simulink library "libc_parts_valves"  (R2015b)
settings: Solver=FixedStepDiscrete  StartTime=0.0  StopTime=Inf  FixedStep=0.004  RelTol=1e-3
PostLoadFcn:
  | , if any(exist('dsrtsu_mdlpostloadfcn', 'file') == [2, 3, 6]), try dsrtsu_mdlpostloadfcn('Execute', bdroot); catch fprintf('Error in PostLoadFcn (dsrtsu_mdlpostloadfcn) for model "%s":\n %s\n', bdroot, lasterr); end, end,
undefined symbols (not defined in the file or in its folder): den, num
undefined symbols (not defined in the file): tA
libraries: libc_parts_valves x9, simulink x6, libc_extended_basics x2, PMC_lib x1
settings Model: DSRTSU_INTERNAL_RTI_VER=470  DSRTSU_INTERNAL_RTI_TYPE=rti1007  DSRTSU_INTERNAL_RTIFPGA=60  Creator=Falkenhahn  LastModifiedBy=Falkenhahn
settings DataIOCC: SaveFormat=Array
settings OptimizationCC: BlockReduction=off  OptimizeBlockIOStorage=off  BufferReuse=off  GlobalBufferReuse=off  ExpressionFolding=off  LocalBlockOutputs=off
settings DebuggingCC: UnderspecifiedInitializationDetection=Classic  MergeDetectMultiDrivingBlocksExec=none  SolverPrmCheckMsg=warning
settings HardwareCC: ProdBitPerPointer=32  ProdLargestAtomicFloat=None  ProdEndianess=BigEndian  ProdWordSize=32  ProdHWDeviceType=Generic->Custom  TargetIntDivRoundTo=Zero  TargetEndianess=BigEndian  TargetHWDeviceType=Generic->Custom
settings RTWCC: SystemTargetFile=rti1007.tlc  MakeCommand=make_rti  TemplateMakefile=rti1007.tmf  Description=dSPACE DS1007 Hardware Platform
settings STFCustomTargetCC: ParMdlRefBuildCompliant=on  ConcurrentExecutionCompliant=off  MatFileLogging=on  SystemTargetFile=rti1007.tlc
settings GRTTargetCC: CompOptLevelCompliant=off  ConcurrentExecutionCompliant=off  GeneratePreprocessorConditionals=Disable all  CombineOutputUpdateFcns=off  GRTInterface=on  UseToolchainInfoCompliant=off  ExtModeMexFile=noextcomm
settings ConfigComp: CovModelRefEnable=Off

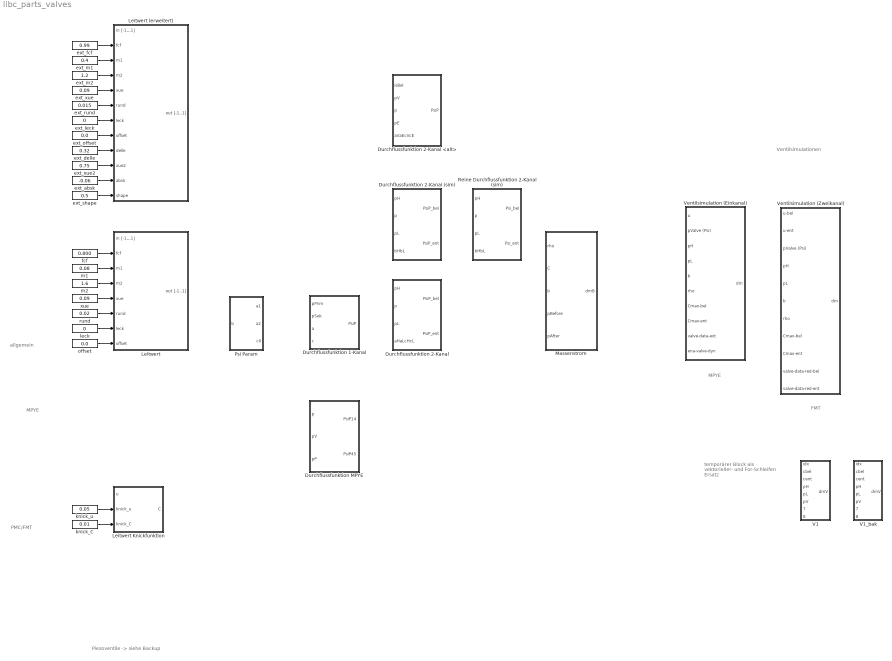
== system libc_parts_valves ==
  note: temporärer Block als
      | vektorieller- und For-Schleifen
      | Ersatz
  note: MPYE
  note: allgemein
  note: MPYE
  note: Piezoventile -> siehe Backup
  note: PMC/FMT
  note: Ventilsimulationen
  note: FMT
  Durchflussfunktion 1-Kanal : Subsystem
      settings: AttributesFormatString=gebrochenrational
  Durchflussfunktion 2-Kanal : Subsystem
      settings: AttributesFormatString=gebrochenrational
  Durchflussfunktion 2-Kanal (sim) : Subsystem
      settings: AttributesFormatString=|
      | Wurzelfunktion
      | (nicht geeignet für Ventilinvertierung)
  Durchflussfunktion 2-Kanal <alt> : Subsystem
      settings: AttributesFormatString=gebrochenrational
  Durchflussfunktion MPYE : Subsystem
      settings: AttributesFormatString=|
      | gebrochenrational
      | kanalweise mit b=0.3
  Leitwert : Subsystem  mask{invertcomp=on}
      mask prompts: invertcomp "Invertierter Leitwert"
      mask help: Leitwertberechnung
      settings: AttributesFormatString=|
      | inv: Cn --> u (on)
      | hin: u --> Cn (off)
      | Invertiert: %<invertcomp>
  Leitwert (erweitert) : Subsystem  mask{invertcomp=on}
      mask prompts: invertcomp "Invertierter Leitwert"
      mask help: Leitwertberechnung
      settings: AttributesFormatString=|
      | inv: Cn --> u (on)
      | hin: u --> Cn (off)
      | Invertiert: %<invertcomp>
  Leitwert Knickfunktion : MATLAB Function  TreatAsAtomicUnit=on
      settings: AttributesFormatString=|
      | u (0..1) -> C (0..1)
      | vertausche knick_u
      | und knick_C-Parameter
      | zur Berechnung der
      | Invertierung
  Massenstrom : Subsystem
  Psi Param : Subsystem
      settings: AttributesFormatString=sqrt -> geb-rat
  Reine Durchflussfunktion 2-Kanal (sim) : Subsystem
      settings: AttributesFormatString=Wurzelfunktion
  V1 : Subsystem
  V1_bak : Subsystem
  Ventilsimulation (Einkanal) : Subsystem
      settings: AttributesFormatString=|
      | mit Wurzelfunktion
      | nicht für Invertierung geeignet
  Ventilsimulation (Zweikanal) : Subsystem
      settings: AttributesFormatString=|
      | mit Wurzelfunktion
      | nicht für Invertierung geeignet
      | 2-Kanal (reduzierte valve-data, ohne valve_dyn)
  ext_absk : Constant  Value=-0.06
  ext_delle : Constant  Value=0.32
  ext_fcf : Constant  Value=0.99
  ext_leck : Constant  Value=0
  ext_m1 : Constant  Value=0.4
  ext_m2 : Constant  Value=1.2
  ext_offset : Constant  Value=0.0
  ext_rund : Constant  Value=0.015
  ext_shape : Constant  Value=0.5
  ext_xue : Constant  Value=0.09
  ext_xue2 : Constant  Value=0.75
  fcf : Constant  Value=0.800
  knick_C : Constant  Value=0.01
  knick_u : Constant  Value=0.05
  leck : Constant  Value=0
  m1 : Constant  Value=0.08
  m2 : Constant  Value=1.6
  offset : Constant  Value=0.0
  rund : Constant  Value=0.02
  xue : Constant  Value=0.09
  wires:
  m1/1 -> Leitwert/3(m1)
  fcf/1 -> Leitwert/2(fcf)
  offset/1 -> Leitwert/8(offset)
  rund/1 -> Leitwert/6(rund)
  m2/1 -> Leitwert/4(m2)
  xue/1 -> Leitwert/5(xue)
  leck/1 -> Leitwert/7(leck)
  ext_m1/1 -> Leitwert (erweitert)/3(m1)
  ext_fcf/1 -> Leitwert (erweitert)/2(fcf)
  ext_offset/1 -> Leitwert (erweitert)/8(offset)
  ext_rund/1 -> Leitwert (erweitert)/6(rund)
  ext_m2/1 -> Leitwert (erweitert)/4(m2)
  ext_xue/1 -> Leitwert (erweitert)/5(xue)
  ext_leck/1 -> Leitwert (erweitert)/7(leck)
  ext_delle/1 -> Leitwert (erweitert)/9(delle)
  ext_xue2/1 -> Leitwert (erweitert)/10(xue2)
  ext_absk/1 -> Leitwert (erweitert)/11(absk)
  ext_shape/1 -> Leitwert (erweitert)/12(shape)
  knick_u/1 -> Leitwert Knickfunktion/2(knick_u)
  knick_C/1 -> Leitwert Knickfunktion/3(knick_C)

== system libc_parts_valves/Durchflussfunktion 1-Kanal ==
  pPrim : Inport
  pSek : Inport  Port=2
  a : Inport  Port=3
  c : Inport  Port=4
  Durchflussfunktion 1 : MATLAB Function  TreatAsAtomicUnit=on
      settings: AttributesFormatString=gebrochenrational
  PsiP : Outport
  wires:
  pSek/1 -> Durchflussfunktion 1/2(pSek)
  a/1 -> Durchflussfunktion 1/3(a)
  pPrim/1 -> Durchflussfunktion 1/1(pPrim)
  Durchflussfunktion 1/1(PsiP) -> PsiP/1
  c/1 -> Durchflussfunktion 1/4(c)

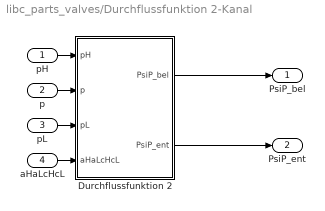
== system libc_parts_valves/Durchflussfunktion 2-Kanal ==
  pH : Inport
  p : Inport  Port=2
  pL : Inport  Port=3
  aHaLcHcL : Inport  Port=4
  Durchflussfunktion 2 : MATLAB Function  TreatAsAtomicUnit=on
      settings: AttributesFormatString=gebrochenrational
  PsiP_bel : Outport
  PsiP_ent : Outport  Port=2
  wires:
  pH/1 -> Durchflussfunktion 2/1(pH)
  pL/1 -> Durchflussfunktion 2/3(pL)
  p/1 -> Durchflussfunktion 2/2(p)
  aHaLcHcL/1 -> Durchflussfunktion 2/4(aHaLcHcL)
  Durchflussfunktion 2/1(PsiP_bel) -> PsiP_bel/1
  Durchflussfunktion 2/2(PsiP_ent) -> PsiP_ent/1

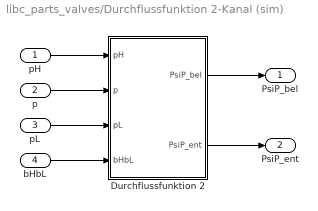
== system libc_parts_valves/Durchflussfunktion 2-Kanal (sim) ==
  pH : Inport
  p : Inport  Port=2
  pL : Inport  Port=3
  bHbL : Inport  Port=4
  Durchflussfunktion 2 : MATLAB Function  TreatAsAtomicUnit=on
      settings: AttributesFormatString=Wurzelfunktion
  PsiP_bel : Outport
  PsiP_ent : Outport  Port=2
  wires:
  Durchflussfunktion 2/2(PsiP_ent) -> PsiP_ent/1
  Durchflussfunktion 2/1(PsiP_bel) -> PsiP_bel/1
  bHbL/1 -> Durchflussfunktion 2/4(bHbL)
  p/1 -> Durchflussfunktion 2/2(p)
  pL/1 -> Durchflussfunktion 2/3(pL)
  pH/1 -> Durchflussfunktion 2/1(pH)

== system libc_parts_valves/Durchflussfunktion 2-Kanal <alt> ==
  isBel : Inport
  pV : Inport  Port=2
  p : Inport  Port=3
  pE : Inport  Port=4
  aVaEcVcE : Inport  Port=5
  Durchflussfunktion 2 : MATLAB Function  TreatAsAtomicUnit=on
      settings: AttributesFormatString=gebrochenrational
  PsiP : Outport
  wires:
  isBel/1 -> Durchflussfunktion 2/1(isBel)
  pV/1 -> Durchflussfunktion 2/2(pV)
  pE/1 -> Durchflussfunktion 2/4(pE)
  p/1 -> Durchflussfunktion 2/3(p)
  aVaEcVcE/1 -> Durchflussfunktion 2/5(aVaEcVcE)
  Durchflussfunktion 2/1(PsiP) -> PsiP/1

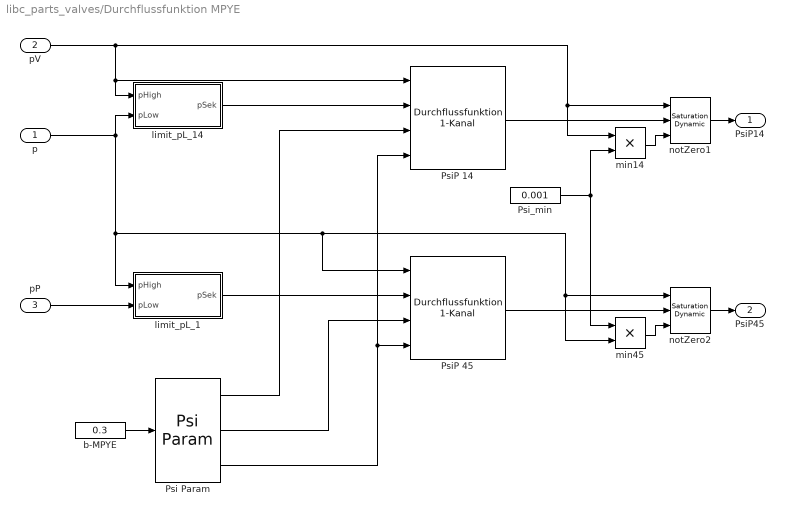
== system libc_parts_valves/Durchflussfunktion MPYE ==
  p : Inport
  pV : Inport  Port=2
  pP : Inport  Port=3
  Psi Param : libc_parts_valves/Psi Param
      settings: AttributesFormatString=sqrt -> geb-rat
  PsiP 14 : libc_parts_valves/Durchflussfunktion 1-Kanal
      settings: AttributesFormatString=gebrochenrational
  PsiP 45 : libc_parts_valves/Durchflussfunktion 1-Kanal
      settings: AttributesFormatString=gebrochenrational
  Psi_min : Constant  Value=0.001
  b-MPYE : Constant  Value=0.3
  limit_pL_1 : MATLAB Function  TreatAsAtomicUnit=on
  limit_pL_14 : MATLAB Function  TreatAsAtomicUnit=on
  min14 : Product  RndMeth=Zero
  min45 : Product  RndMeth=Zero
  notZero1 : simulink/Discontinuities/Saturation Dynamic  OutMin=[]  OutMax=[]  OutDataTypeStr=Inherit: Same as second input  OutDataType=fixdt(1, 16)  OutScaling=2^-10  DoSatur=off
  notZero2 : simulink/Discontinuities/Saturation Dynamic  OutMin=[]  OutMax=[]  OutDataTypeStr=Inherit: Same as second input  OutDataType=fixdt(1, 16)  OutScaling=2^-10  DoSatur=off
  PsiP14 : Outport
  PsiP45 : Outport  Port=2
  wires:
  Psi_min/1 -> min45/1, min14/2
  min45/1 -> notZero2/3
  min14/1 -> notZero1/3
  notZero2/1 -> PsiP45/1
  PsiP 45/1 -> notZero2/2
  notZero1/1 -> PsiP14/1
  PsiP 14/1 -> notZero1/2
  limit_pL_1/1(pSek) -> PsiP 45/2
  limit_pL_14/1(pSek) -> PsiP 14/2
  p/1 -> limit_pL_1/1(pHigh), PsiP 45/1, notZero2/1, min45/2, limit_pL_14/2(pLow)
  pP/1 -> limit_pL_1/2(pLow)
  pV/1 -> notZero1/1, min14/1, PsiP 14/1, limit_pL_14/1(pHigh)
  Psi Param/1 -> PsiP 14/3
  Psi Param/2 -> PsiP 45/3
  Psi Param/3 -> PsiP 14/4, PsiP 45/4
  b-MPYE/1 -> Psi Param/1

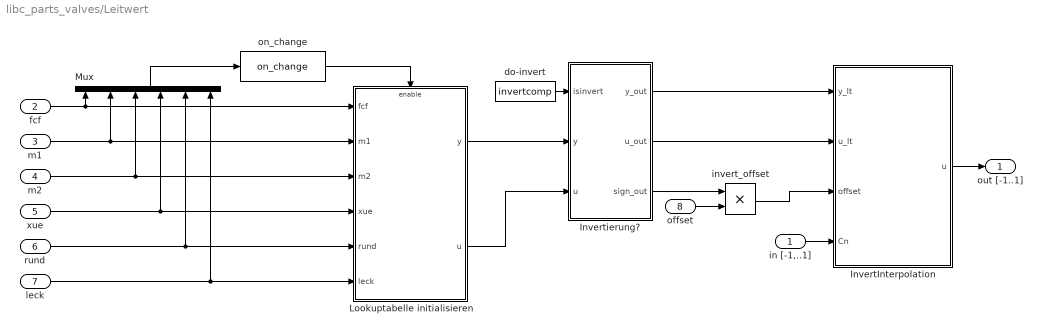
== system libc_parts_valves/Leitwert ==
  in [-1,..1] : Inport
  fcf : Inport  Port=2
  m1 : Inport  Port=3
  m2 : Inport  Port=4
  xue : Inport  Port=5
  rund : Inport  Port=6
  leck : Inport  Port=7
  offset : Inport  Port=8
  InvertInterpolation : MATLAB Function  TreatAsAtomicUnit=on
      settings: AttributesFormatString=|
      | 2 Versionen:
      | alt (PLC-kompatibel)
      | neu (interp1)
  Invertierung? : MATLAB Function  TreatAsAtomicUnit=on
  Lookuptabelle initialisieren : Subsystem  TreatAsAtomicUnit=on
      settings: AttributesFormatString=|
      | 2 Versionen:
      | alt (PLC-kompatibel, mit/ohne Fehler)
      | neu (schnell)
  Mux : Mux  Inputs=6
  do-invert : Constant  Value=invertcomp
  invert_offset : Product
  on_change : libc_extended_basics/on_change  IC=-1
  out [-1..1] : Outport
  wires:
  leck/1 -> Mux/6, Lookuptabelle initialisieren/6(leck)
  Lookuptabelle initialisieren/2(u) -> Invertierung?/3(u)
  offset/1 -> invert_offset/2
  m1/1 -> Mux/2, Lookuptabelle initialisieren/2(m1)
  m2/1 -> Mux/3, Lookuptabelle initialisieren/3(m2)
  rund/1 -> Mux/5, Lookuptabelle initialisieren/5(rund)
  xue/1 -> Mux/4, Lookuptabelle initialisieren/4(xue)
  Lookuptabelle initialisieren/1(y) -> Invertierung?/2(y)
  fcf/1 -> Mux/1, Lookuptabelle initialisieren/1(fcf)
  InvertInterpolation/1(u) -> out [-1..1]/1
  in [-1,..1]/1 -> InvertInterpolation/4(Cn)
  on_change/1 -> Lookuptabelle initialisieren/Enable
  Mux/1 -> on_change/1
  Invertierung?/2(u_out) -> InvertInterpolation/2(u_lt)
  Invertierung?/1(y_out) -> InvertInterpolation/1(y_lt)
  invert_offset/1 -> InvertInterpolation/3(offset)
  Invertierung?/3(sign_out) -> invert_offset/1
  do-invert/1 -> Invertierung?/1(isinvert)

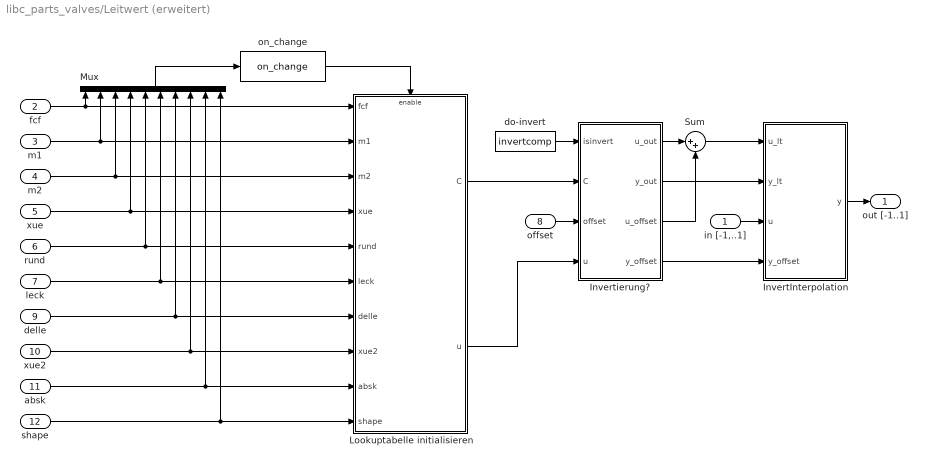
== system libc_parts_valves/Leitwert (erweitert) ==
  in [-1,..1] : Inport
  fcf : Inport  Port=2
  m1 : Inport  Port=3
  m2 : Inport  Port=4
  xue : Inport  Port=5
  rund : Inport  Port=6
  leck : Inport  Port=7
  offset : Inport  Port=8
  delle : Inport  Port=9
  xue2 : Inport  Port=10
  absk : Inport  Port=11
  shape : Inport  Port=12
  InvertInterpolation : MATLAB Function  TreatAsAtomicUnit=on
      settings: AttributesFormatString=|
      | 2 Versionen:
      | alt (PLC-kompatibel)
      | neu (interp1)
  Invertierung? : MATLAB Function  TreatAsAtomicUnit=on
  Lookuptabelle initialisieren : Subsystem  TreatAsAtomicUnit=on
      settings: AttributesFormatString=|
      | 2 Versionen:
      | alt (PLC-kompatibel, mit/ohne Fehler)
      | neu (schnell)
  Mux : Mux  Inputs=10
  Sum : Sum  Inputs=|++
  do-invert : Constant  Value=invertcomp
  on_change : libc_extended_basics/on_change  IC=-1
  out [-1..1] : Outport
  wires:
  Invertierung?/4(y_offset) -> InvertInterpolation/4(y_offset)
  Lookuptabelle initialisieren/2(u) -> Invertierung?/4(u)
  Lookuptabelle initialisieren/1(C) -> Invertierung?/2(C)
  shape/1 -> Lookuptabelle initialisieren/10(shape), Mux/10
  absk/1 -> Lookuptabelle initialisieren/9(absk), Mux/9
  xue2/1 -> Lookuptabelle initialisieren/8(xue2), Mux/8
  delle/1 -> Lookuptabelle initialisieren/7(delle), Mux/7
  leck/1 -> Lookuptabelle initialisieren/6(leck), Mux/6
  offset/1 -> Invertierung?/3(offset)
  m1/1 -> Lookuptabelle initialisieren/2(m1), Mux/2
  m2/1 -> Lookuptabelle initialisieren/3(m2), Mux/3
  rund/1 -> Lookuptabelle initialisieren/5(rund), Mux/5
  xue/1 -> Lookuptabelle initialisieren/4(xue), Mux/4
  fcf/1 -> Mux/1, Lookuptabelle initialisieren/1(fcf)
  in [-1,..1]/1 -> InvertInterpolation/3(u)
  on_change/1 -> Lookuptabelle initialisieren/Enable
  Mux/1 -> on_change/1
  do-invert/1 -> Invertierung?/1(isinvert)
  Invertierung?/1(u_out) -> Sum/1
  Sum/1 -> InvertInterpolation/1(u_lt)
  Invertierung?/2(y_out) -> InvertInterpolation/2(y_lt)
  Invertierung?/3(u_offset) -> Sum/2
  InvertInterpolation/1(y) -> out [-1..1]/1

== system libc_parts_valves/Massenstrom ==
  rho : Inport
  C : Inport  Port=2
  b : Inport  Port=3
  pBefore : Inport  Port=4
  pAfter : Inport  Port=5
  Massenstrom : MATLAB Function  TreatAsAtomicUnit=on
  dmB : Outport
  wires:
  pBefore/1 -> Massenstrom/4(pBefore)
  pAfter/1 -> Massenstrom/5(pAfter)
  C/1 -> Massenstrom/2(parC)
  b/1 -> Massenstrom/3(parb)
  Massenstrom/1(mBdot) -> dmB/1
  rho/1 -> Massenstrom/1(parrho)

== system libc_parts_valves/Psi Param ==
  b : Inport
  b-auto : MATLAB Function  TreatAsAtomicUnit=on
  a1 : Outport
  a2 : Outport  Port=2
  c0 : Outport  Port=3
  wires:
  b/1 -> b-auto/1(b)
  b-auto/1(a1) -> a1/1
  b-auto/3(c0) -> c0/1
  b-auto/2(a2) -> a2/1

== system libc_parts_valves/Reine Durchflussfunktion 2-Kanal (sim) ==
  pH : Inport
  p : Inport  Port=2
  pL : Inport  Port=3
  bHbL : Inport  Port=4
  Durchflussfunktion 2 : MATLAB Function  TreatAsAtomicUnit=on
      settings: AttributesFormatString=Wurzelfunktion
  Psi_bel : Outport
  Psi_ent : Outport  Port=2
  wires:
  pH/1 -> Durchflussfunktion 2/1(pH)
  pL/1 -> Durchflussfunktion 2/3(pL)
  p/1 -> Durchflussfunktion 2/2(p)
  bHbL/1 -> Durchflussfunktion 2/4(bHbL)
  Durchflussfunktion 2/1(Psi_bel) -> Psi_bel/1
  Durchflussfunktion 2/2(Psi_ent) -> Psi_ent/1

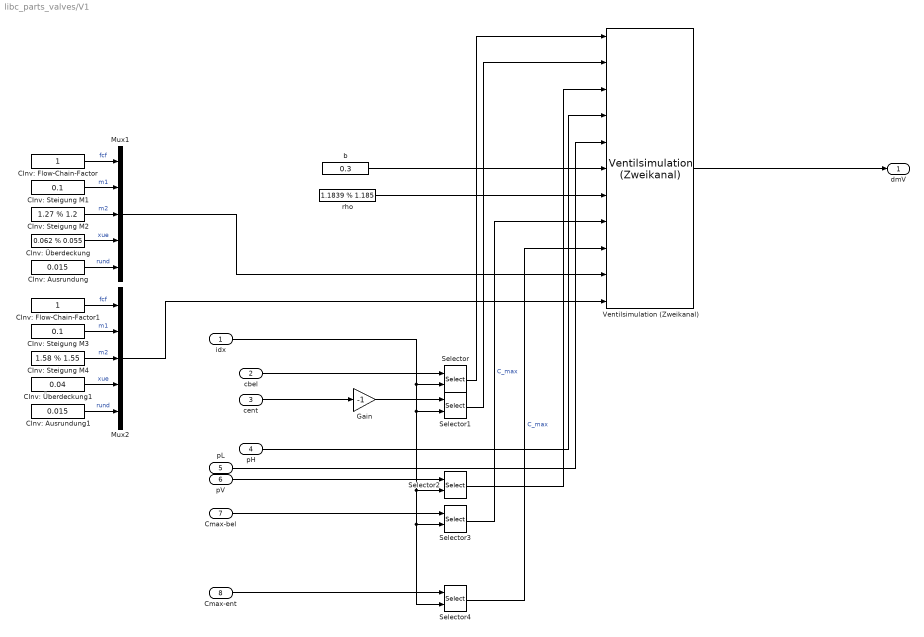
== system libc_parts_valves/V1 ==
  idx : Inport
  cbel : Inport  Port=2
  cent : Inport  Port=3
  pH : Inport  Port=4
  pL : Inport  Port=5
  pV : Inport  Port=6
  Cmax-bel : Inport  Port=7
  Cmax-ent : Inport  Port=8
  CInv: Ausrundung : Constant  Value=0.015
  CInv: Ausrundung1 : Constant  Value=0.015
  CInv: Flow-Chain-Factor : Constant
  CInv: Flow-Chain-Factor1 : Constant
  CInv: Steigung M1 : Constant  Value=0.1
  CInv: Steigung M2 : Constant  Value=1.27 % 1.2
  CInv: Steigung M3 : Constant  Value=0.1
  CInv: Steigung M4 : Constant  Value=1.58 % 1.55
  CInv: Überdeckung : Constant  Value=0.062 % 0.055
  CInv: Überdeckung1 : Constant  Value=0.04
  Gain : Gain  Gain=-1
      settings: AttributesFormatString=|
      | Massenstrom-Block
      | benötigt negativen
      | Entlüftungshub
  Mux1 : Mux  Inputs=5
  Mux2 : Mux  Inputs=5
  Selector{,1..4} (5 alike) : Selector  InputPortWidth=9  IndexOptions=Index vector (port)  Indices=1  OutputSizes=1
  Ventilsimulation (Zweikanal) : libc_parts_valves/Ventilsimulation (Zweikanal)
      settings: AttributesFormatString=|
      | mit Wurzelfunktion
      | nicht für Invertierung geeignet
      | 2-Kanal (reduzierte valve-data, ohne valve_dyn)
  b : Constant  Value=0.3
      settings: AttributesFormatString=0.3
  rho : Constant  Value=1.1839 % 1.185
  dmV : Outport
  wires:
  idx/1 -> Selector1/2, Selector2/2, Selector4/2, Selector3/2, Selector/2
  Cmax-ent/1 -> Selector4/1
  Cmax-bel/1 -> Selector3/1
  Selector/1 -> Ventilsimulation (Zweikanal)/1
  Selector2/1 -> Ventilsimulation (Zweikanal)/3
  Selector3/1 -> Ventilsimulation (Zweikanal)/8  "C_max"
  Selector4/1 -> Ventilsimulation (Zweikanal)/9  "C_max"
  pL/1 -> Ventilsimulation (Zweikanal)/5
  pH/1 -> Ventilsimulation (Zweikanal)/4
  pV/1 -> Selector2/1
  cbel/1 -> Selector/1
  Selector1/1 -> Ventilsimulation (Zweikanal)/2
  Gain/1 -> Selector1/1
  cent/1 -> Gain/1
  rho/1 -> Ventilsimulation (Zweikanal)/7
  b/1 -> Ventilsimulation (Zweikanal)/6
  CInv: Flow-Chain-Factor/1 -> Mux1/1  "fcf"
  CInv: Ausrundung/1 -> Mux1/5  "rund"
  CInv: Steigung M2/1 -> Mux1/3  "m2"
  CInv: Steigung M1/1 -> Mux1/2  "m1"
  CInv: Überdeckung/1 -> Mux1/4  "xue"
  Mux1/1 -> Ventilsimulation (Zweikanal)/10
  CInv: Flow-Chain-Factor1/1 -> Mux2/1  "fcf"
  CInv: Ausrundung1/1 -> Mux2/5  "rund"
  CInv: Steigung M4/1 -> Mux2/3  "m2"
  CInv: Steigung M3/1 -> Mux2/2  "m1"
  CInv: Überdeckung1/1 -> Mux2/4  "xue"
  Mux2/1 -> Ventilsimulation (Zweikanal)/11
  Ventilsimulation (Zweikanal)/1 -> dmV/1

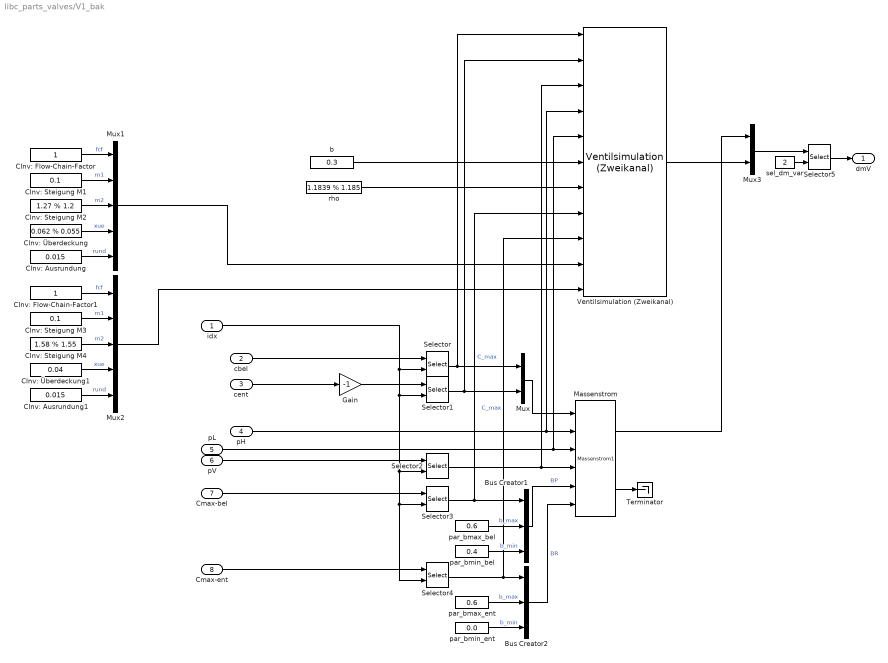
== system libc_parts_valves/V1_bak ==
  idx : Inport
  cbel : Inport  Port=2
  cent : Inport  Port=3
  pH : Inport  Port=4
  pL : Inport  Port=5
  pV : Inport  Port=6
  Cmax-bel : Inport  Port=7
  Cmax-ent : Inport  Port=8
  Bus Creator1 : BusCreator  Inputs=3
  Bus Creator2 : BusCreator  Inputs=3
  CInv: Ausrundung : Constant  Value=0.015
  CInv: Ausrundung1 : Constant  Value=0.015
  CInv: Flow-Chain-Factor : Constant
  CInv: Flow-Chain-Factor1 : Constant
  CInv: Steigung M1 : Constant  Value=0.1
  CInv: Steigung M2 : Constant  Value=1.27 % 1.2
  CInv: Steigung M3 : Constant  Value=0.1
  CInv: Steigung M4 : Constant  Value=1.58 % 1.55
  CInv: Überdeckung : Constant  Value=0.062 % 0.055
  CInv: Überdeckung1 : Constant  Value=0.04
  Gain : Gain  Gain=-1
      settings: AttributesFormatString=|
      | Massenstrom-Block
      | benötigt negativen
      | Entlüftungshub
  Massenstrom : PMC_lib/Durchflussfunktion/Massenstrom1
  Mux : Mux  Inputs=2
  Mux1 : Mux  Inputs=5
  Mux2 : Mux  Inputs=5
  Mux3 : Mux  Inputs=2
  Selector{,1..4} (5 alike) : Selector  InputPortWidth=9  IndexOptions=Index vector (port)  Indices=1  OutputSizes=1
  Selector5 : Selector  InputPortWidth=2  IndexOptions=Index vector (port)  Indices=1  OutputSizes=1
  Terminator : Terminator
  Ventilsimulation (Zweikanal) : libc_parts_valves/Ventilsimulation (Zweikanal)
      settings: AttributesFormatString=|
      | mit Wurzelfunktion
      | nicht für Invertierung geeignet
      | 2-Kanal (reduzierte valve-data, ohne valve_dyn)
  b : Constant  Value=0.3
      settings: AttributesFormatString=0.3
  par_bmax_bel : Constant  Value=0.6
  par_bmax_ent : Constant  Value=0.6
  par_bmin_bel : Constant  Value=0.4
  par_bmin_ent : Constant  Value=0.0
  rho : Constant  Value=1.1839 % 1.185
  sel_dm_var : Constant  Value=2
  dmV : Outport
  wires:
  sel_dm_var/1 -> Selector5/2
  Selector5/1 -> dmV/1
  Mux3/1 -> Selector5/1
  Ventilsimulation (Zweikanal)/1 -> Mux3/2
  Mux2/1 -> Ventilsimulation (Zweikanal)/11
  CInv: Überdeckung1/1 -> Mux2/4  "xue"
  CInv: Steigung M3/1 -> Mux2/2  "m1"
  CInv: Steigung M4/1 -> Mux2/3  "m2"
  CInv: Ausrundung1/1 -> Mux2/5  "rund"
  CInv: Flow-Chain-Factor1/1 -> Mux2/1  "fcf"
  Mux1/1 -> Ventilsimulation (Zweikanal)/10
  CInv: Überdeckung/1 -> Mux1/4  "xue"
  CInv: Steigung M1/1 -> Mux1/2  "m1"
  CInv: Steigung M2/1 -> Mux1/3  "m2"
  CInv: Ausrundung/1 -> Mux1/5  "rund"
  CInv: Flow-Chain-Factor/1 -> Mux1/1  "fcf"
  b/1 -> Ventilsimulation (Zweikanal)/6
  rho/1 -> Ventilsimulation (Zweikanal)/7
  cent/1 -> Gain/1
  Gain/1 -> Selector1/1
  Selector1/1 -> Mux/2, Ventilsimulation (Zweikanal)/2
  cbel/1 -> Selector/1
  pV/1 -> Selector2/1
  pH/1 -> Massenstrom/2, Ventilsimulation (Zweikanal)/4
  pL/1 -> Massenstrom/3, Ventilsimulation (Zweikanal)/5
  Massenstrom/2 -> Terminator/1
  Mux/1 -> Massenstrom/1
  par_bmin_ent/1 -> Bus Creator2/3  "b_min"
  Selector4/1 -> Bus Creator2/1, Ventilsimulation (Zweikanal)/9  "C_max"
  par_bmin_bel/1 -> Bus Creator1/3  "b_min"
  par_bmax_ent/1 -> Bus Creator2/2  "b_max"
  par_bmax_bel/1 -> Bus Creator1/2  "b_max"
  Bus Creator2/1 -> Massenstrom/6  "BR"
  Selector3/1 -> Bus Creator1/1, Ventilsimulation (Zweikanal)/8  "C_max"
  Selector2/1 -> Massenstrom/4, Ventilsimulation (Zweikanal)/3
  Selector/1 -> Mux/1, Ventilsimulation (Zweikanal)/1
  Massenstrom/1 -> Mux3/1
  Bus Creator1/1 -> Massenstrom/5  "BP"
  Cmax-bel/1 -> Selector3/1
  Cmax-ent/1 -> Selector4/1
  idx/1 -> Selector/2, Selector3/2, Selector4/2, Selector2/2, Selector1/2

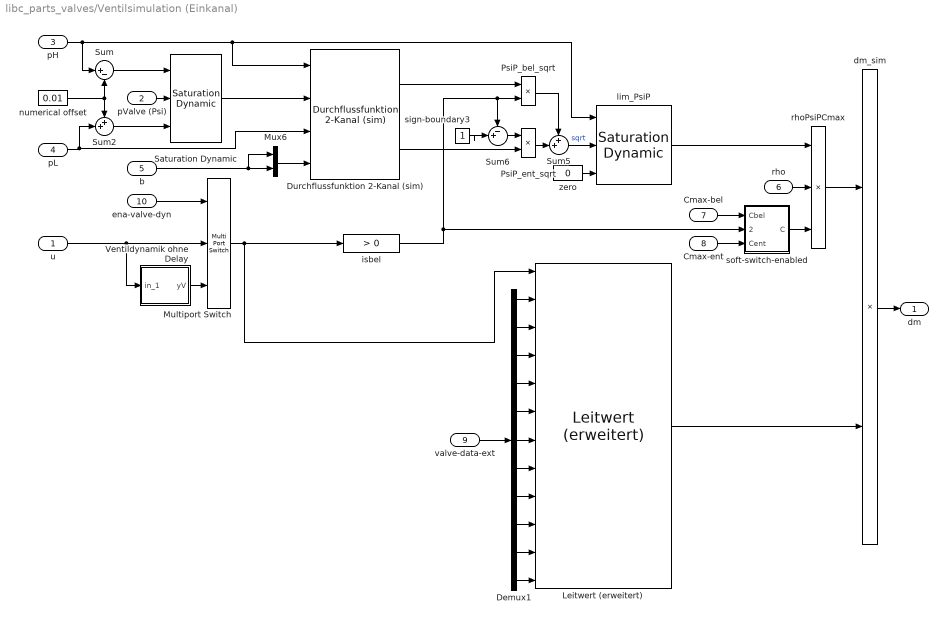
== system libc_parts_valves/Ventilsimulation (Einkanal) ==
  u : Inport
  pValve (Psi) : Inport  Port=2
  pH : Inport  Port=3
  pL : Inport  Port=4
  b : Inport  Port=5
  rho : Inport  Port=6
  Cmax-bel : Inport  Port=7
  Cmax-ent : Inport  Port=8
  valve-data-ext : Inport  Port=9
  ena-valve-dyn : Inport  Port=10
  Demux1 : Demux  Outputs=11
  Durchflussfunktion 2-Kanal (sim) : libc_parts_valves/Durchflussfunktion 2-Kanal (sim)
      settings: AttributesFormatString=|
      | Wurzelfunktion
      | (nicht geeignet für Ventilinvertierung)
  Leitwert (erweitert) : libc_parts_valves/Leitwert (erweitert)  invertcomp=off
      settings: AttributesFormatString=|
      | inv: Cn --> u (on)
      | hin: u --> Cn (off)
      | Invertiert: %<invertcomp>
  Multiport Switch : MultiPortSwitch  DataPortOrder=Zero-based contiguous  Inputs=2
  Mux6 : Mux  Inputs=2
  PsiP_bel_sqrt : Product
  PsiP_ent_sqrt : Product
  Saturation Dynamic : simulink/Discontinuities/Saturation Dynamic  OutMin=[]  OutMax=[]  OutDataTypeStr=Inherit: Same as second input  OutDataType=fixdt(1, 16)  OutScaling=2^-10  DoSatur=off
  Sum : Sum  Inputs=|+-
  Sum2 : Sum  Inputs=++|
  Sum5 : Sum  Inputs=++|
  Sum6 : Sum  Inputs=-+|
  Ventildynamik ohne Delay : Subsystem  mask(Ventilverzoegerung){wv=200*2*pi, dv=0.6, grenze=0.3, offset=0}
      mask prompts: wv "Eigenfreqenz"; dv "Daempfung"; grenze "Begrenzung"
      mask help: System 2. Ord. mit Begrenzung
      mask init:
      | [num,den]=ord2(wv,dv); t=0:0.5/wv:15/wv; u=0*t+1; u(1)=0;  y=lsim(num,den,u,t);
      mask Display: plot([0:0.1:1],[0 0.05 0.5 0.9 1.0 0.93 0.93 0.97 0.95 0.95 0.95]);
  dm_sim : Product  Inputs=**
  isbel : simulink/Logic and Bit Operations/Compare To Zero  relop=>  OutDataTypeStr=boolean
      settings: AttributesFormatString=|
      | Beim Beobachter macht es keinen Unterschied,
      | ob weicher oder harter Übergang, da u dort
      | immer 0 (klein) ist, jedoch nicht durch 0 dividiert wird
  lim_PsiP : simulink/Discontinuities/Saturation Dynamic  OutMin=[]  OutMax=[]  OutDataTypeStr=Inherit: Same as second input  OutDataType=fixdt(1, 16)  OutScaling=2^-10  DoSatur=off
      settings: AttributesFormatString=|
      | Unterer Schranke
      | im Entlüften nicht
      | pE sondern 0
  numerical offset : Constant  Value=0.01
  rhoPsiPCmax : Product  Inputs=***
  sign-boundary3 : Constant
  soft-switch-enabled : MATLAB Function  TreatAsAtomicUnit=on
  zero : Constant  Value=0
  dm : Outport
  wires:
  Sum5/1 -> lim_PsiP/2  "sqrt"
  PsiP_ent_sqrt/1 -> Sum5/2
  sign-boundary3/1 -> Sum6/2
  Sum6/1 -> PsiP_ent_sqrt/1
  Durchflussfunktion 2-Kanal (sim)/2 -> PsiP_ent_sqrt/2
  Durchflussfunktion 2-Kanal (sim)/1 -> PsiP_bel_sqrt/1
  PsiP_bel_sqrt/1 -> Sum5/1
  Mux6/1 -> Durchflussfunktion 2-Kanal (sim)/4
  b/1 -> Mux6/2, Mux6/1
  isbel/1 -> soft-switch-enabled/2(alpha), PsiP_bel_sqrt/2, Sum6/1
  Demux1/11 -> Leitwert (erweitert)/12
  Demux1/8 -> Leitwert (erweitert)/9
  Demux1/10 -> Leitwert (erweitert)/11
  Demux1/9 -> Leitwert (erweitert)/10
  ena-valve-dyn/1 -> Multiport Switch/1
  zero/1 -> lim_PsiP/3
  Cmax-ent/1 -> soft-switch-enabled/3(Cent)
  soft-switch-enabled/1(C) -> rhoPsiPCmax/3
  Ventildynamik ohne Delay/1(yV) -> Multiport Switch/3
  Cmax-bel/1 -> soft-switch-enabled/1(Cbel)
  rho/1 -> rhoPsiPCmax/2
  pH/1 -> lim_PsiP/1, Durchflussfunktion 2-Kanal (sim)/1, Sum/1
  Sum/1 -> Saturation Dynamic/1
  lim_PsiP/1 -> rhoPsiPCmax/1
  pValve (Psi)/1 -> Saturation Dynamic/2
  Saturation Dynamic/1 -> Durchflussfunktion 2-Kanal (sim)/2
  rhoPsiPCmax/1 -> dm_sim/1
  pL/1 -> Durchflussfunktion 2-Kanal (sim)/3, Sum2/2
  numerical offset/1 -> Sum/2, Sum2/1
  Sum2/1 -> Saturation Dynamic/3
  valve-data-ext/1 -> Demux1/1
  Multiport Switch/1 -> isbel/1, Leitwert (erweitert)/1
  u/1 -> Ventildynamik ohne Delay/1(in_1), Multiport Switch/2
  Demux1/7 -> Leitwert (erweitert)/8
  Demux1/4 -> Leitwert (erweitert)/5
  Demux1/3 -> Leitwert (erweitert)/4
  Demux1/6 -> Leitwert (erweitert)/7
  Demux1/5 -> Leitwert (erweitert)/6
  Demux1/2 -> Leitwert (erweitert)/3
  Demux1/1 -> Leitwert (erweitert)/2
  Leitwert (erweitert)/1 -> dm_sim/2
  dm_sim/1 -> dm/1

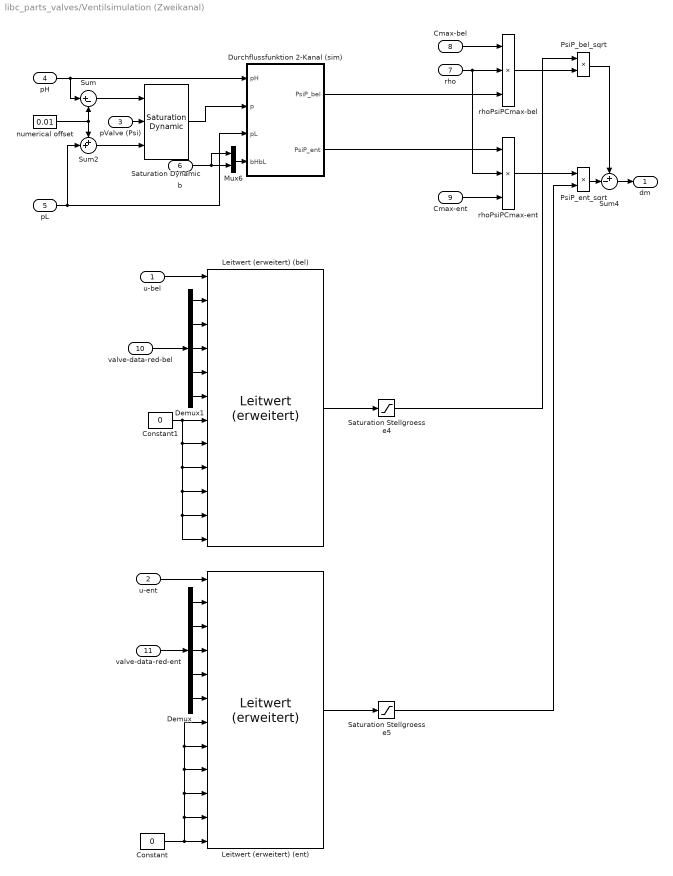
== system libc_parts_valves/Ventilsimulation (Zweikanal) ==
  u-bel : Inport
  u-ent : Inport  Port=2
  pValve (Psi) : Inport  Port=3
  pH : Inport  Port=4
  pL : Inport  Port=5
  b : Inport  Port=6
  rho : Inport  Port=7
  Cmax-bel : Inport  Port=8
  Cmax-ent : Inport  Port=9
  valve-data-red-bel : Inport  Port=10
  valve-data-red-ent : Inport  Port=11
  Constant : Constant  Value=0
  Constant1 : Constant  Value=0
  Demux : Demux  Outputs=5
  Demux1 : Demux  Outputs=5
  Durchflussfunktion 2-Kanal (sim) : Subsystem
      settings: AttributesFormatString=|
      | Wurzelfunktion
      | (nicht geeignet für Ventilinvertierung)
  Leitwert (erweitert) (bel) : libc_parts_valves/Leitwert (erweitert)  invertcomp=off
      settings: AttributesFormatString=|
      | inv: Cn --> u (on)
      | hin: u --> Cn (off)
      | Invertiert: %<invertcomp>
  Leitwert (erweitert) (ent) : libc_parts_valves/Leitwert (erweitert)  invertcomp=off
      settings: AttributesFormatString=|
      | inv: Cn --> u (on)
      | hin: u --> Cn (off)
      | Invertiert: %<invertcomp>
  Mux6 : Mux  Inputs=2
  PsiP_bel_sqrt : Product
  PsiP_ent_sqrt : Product
  Saturation Dynamic : simulink/Discontinuities/Saturation Dynamic  OutMin=[]  OutMax=[]  OutDataTypeStr=Inherit: Same as second input  OutDataType=fixdt(1, 16)  OutScaling=2^-10  DoSatur=off
  Saturation Stellgroesse4 : Saturate  UpperLimit=1  LowerLimit=0
  Saturation Stellgroesse5 : Saturate  UpperLimit=1  LowerLimit=0
  Sum : Sum  Inputs=|+-
  Sum2 : Sum  Inputs=++|
  Sum4 : Sum  Inputs=+-|
  numerical offset : Constant  Value=0.01
  rhoPsiPCmax-bel : Product  Inputs=***
  rhoPsiPCmax-ent : Product  Inputs=***
  dm : Outport
  wires:
  Sum4/1 -> dm/1
  Sum2/1 -> Saturation Dynamic/3
  numerical offset/1 -> Sum2/1, Sum/2
  pL/1 -> Sum2/2, Durchflussfunktion 2-Kanal (sim)/3(pL)
  Saturation Dynamic/1 -> Durchflussfunktion 2-Kanal (sim)/2(p)
  pValve (Psi)/1 -> Saturation Dynamic/2
  Sum/1 -> Saturation Dynamic/1
  pH/1 -> Sum/1, Durchflussfunktion 2-Kanal (sim)/1(pH)
  rho/1 -> rhoPsiPCmax-bel/2, rhoPsiPCmax-ent/2
  b/1 -> Mux6/1, Mux6/2
  Mux6/1 -> Durchflussfunktion 2-Kanal (sim)/4(bHbL)
  PsiP_bel_sqrt/1 -> Sum4/1
  PsiP_ent_sqrt/1 -> Sum4/2
  Durchflussfunktion 2-Kanal (sim)/1(PsiP_bel) -> rhoPsiPCmax-bel/3
  Cmax-bel/1 -> rhoPsiPCmax-bel/1
  Durchflussfunktion 2-Kanal (sim)/2(PsiP_ent) -> rhoPsiPCmax-ent/1
  Cmax-ent/1 -> rhoPsiPCmax-ent/3
  rhoPsiPCmax-ent/1 -> PsiP_ent_sqrt/1
  rhoPsiPCmax-bel/1 -> PsiP_bel_sqrt/2
  Saturation Stellgroesse4/1 -> PsiP_bel_sqrt/1
  Saturation Stellgroesse5/1 -> PsiP_ent_sqrt/2
  Leitwert (erweitert) (bel)/1 -> Saturation Stellgroesse4/1
  Demux/1 -> Leitwert (erweitert) (ent)/2
  Demux/2 -> Leitwert (erweitert) (ent)/3
  Demux/3 -> Leitwert (erweitert) (ent)/4
  Demux/4 -> Leitwert (erweitert) (ent)/5
  Demux/5 -> Leitwert (erweitert) (ent)/6
  Demux1/1 -> Leitwert (erweitert) (bel)/2
  Demux1/2 -> Leitwert (erweitert) (bel)/3
  Demux1/3 -> Leitwert (erweitert) (bel)/4
  Demux1/4 -> Leitwert (erweitert) (bel)/5
  Demux1/5 -> Leitwert (erweitert) (bel)/6
  valve-data-red-bel/1 -> Demux1/1
  valve-data-red-ent/1 -> Demux/1
  u-bel/1 -> Leitwert (erweitert) (bel)/1
  u-ent/1 -> Leitwert (erweitert) (ent)/1
  Constant/1 -> Leitwert (erweitert) (ent)/11, Leitwert (erweitert) (ent)/10, Leitwert (erweitert) (ent)/8, Leitwert (erweitert) (ent)/7, Leitwert (erweitert) (ent)/9, Leitwert (erweitert) (ent)/12
  Constant1/1 -> Leitwert (erweitert) (bel)/8, Leitwert (erweitert) (bel)/9, Leitwert (erweitert) (bel)/11, Leitwert (erweitert) (bel)/12, Leitwert (erweitert) (bel)/10, Leitwert (erweitert) (bel)/7
  Leitwert (erweitert) (ent)/1 -> Saturation Stellgroesse5/1

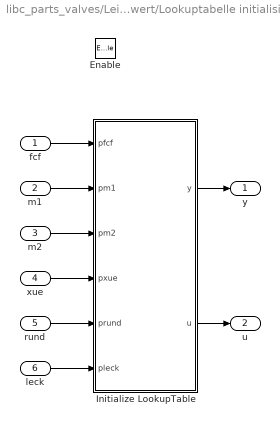
== system libc_parts_valves/Leitwert/Lookuptabelle initialisieren ==
  fcf : Inport
  m1 : Inport  Port=2
  m2 : Inport  Port=3
  xue : Inport  Port=4
  rund : Inport  Port=5
  leck : Inport  Port=6
  Enable : EnablePort
  Initialize LookupTable : MATLAB Function  TreatAsAtomicUnit=on
  y : Outport
  u : Outport  Port=2
  wires:
  Initialize LookupTable/2(u) -> u/1
  Initialize LookupTable/1(y) -> y/1
  leck/1 -> Initialize LookupTable/6(pleck)
  fcf/1 -> Initialize LookupTable/1(pfcf)
  m1/1 -> Initialize LookupTable/2(pm1)
  m2/1 -> Initialize LookupTable/3(pm2)
  rund/1 -> Initialize LookupTable/5(prund)
  xue/1 -> Initialize LookupTable/4(pxue)

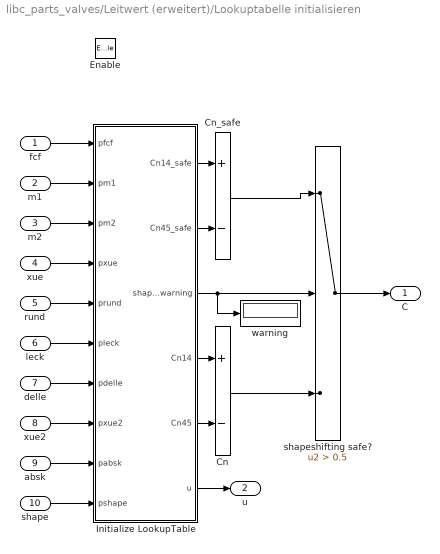
== system libc_parts_valves/Leitwert (erweitert)/Lookuptabelle initialisieren ==
  fcf : Inport
  m1 : Inport  Port=2
  m2 : Inport  Port=3
  xue : Inport  Port=4
  rund : Inport  Port=5
  leck : Inport  Port=6
  delle : Inport  Port=7
  xue2 : Inport  Port=8
  absk : Inport  Port=9
  shape : Inport  Port=10
  Enable : EnablePort
  Cn : Sum  Inputs=+-
  Cn_safe : Sum  Inputs=+-
  Initialize LookupTable : MATLAB Function  TreatAsAtomicUnit=on
  shapeshifting safe? : Switch  Criteria=u2 > Threshold  Threshold=0.5
  warning : Display
  C : Outport
  u : Outport  Port=2
  wires:
  shapeshifting safe?/1 -> C/1
  Initialize LookupTable/3(shapewarning) -> warning/1, shapeshifting safe?/2
  xue2/1 -> Initialize LookupTable/8(pxue2)
  absk/1 -> Initialize LookupTable/9(pabsk)
  shape/1 -> Initialize LookupTable/10(pshape)
  delle/1 -> Initialize LookupTable/7(pdelle)
  Initialize LookupTable/6(u) -> u/1
  leck/1 -> Initialize LookupTable/6(pleck)
  fcf/1 -> Initialize LookupTable/1(pfcf)
  m1/1 -> Initialize LookupTable/2(pm1)
  m2/1 -> Initialize LookupTable/3(pm2)
  rund/1 -> Initialize LookupTable/5(prund)
  xue/1 -> Initialize LookupTable/4(pxue)
  Initialize LookupTable/1(Cn14_safe) -> Cn_safe/1
  Initialize LookupTable/2(Cn45_safe) -> Cn_safe/2
  Cn_safe/1 -> shapeshifting safe?/1
  Initialize LookupTable/4(Cn14) -> Cn/1
  Initialize LookupTable/5(Cn45) -> Cn/2
  Cn/1 -> shapeshifting safe?/3

== system libc_parts_valves/Ventilsimulation (Einkanal)/Ventildynamik ohne Delay ==
  in_1 : Inport
  Saturation : Saturate  UpperLimit=grenze  LowerLimit=-grenze
  Sum : Sum  Inputs=+-  SaturateOnIntegerOverflow=on  InputSameDT=on  OutDataTypeStr=Inherit: Same as first input
  Sum2 : Sum  SaturateOnIntegerOverflow=on  InputSameDT=on  OutDataTypeStr=Inherit: Same as first input
  discrete filter : DiscreteTransferFcn  Numerator=num  Denominator=den  SampleTime=TS  mask{wv=wv, dv=dv, TS=tA}
      mask prompts: wv "Grenzfrequenz (rad/s)"; dv "Dämpfung"; TS "Sample Time"
      mask init:
      | csys = tf(wv^2,[1,2*dv*wv,0]);
      | [nums,dens] = tfdata(csys,'v');
      | [num,den] = tfdata(c2d(csys,TS),'v');
      settings: AttributesFormatString=w²/(s² + 2dws)
      mask Display: dpoly(nums,dens)
  p0 : Constant  Value=offset
  yV : Outport  InitialOutput=0
  wires:
  Sum/1 -> Saturation/1
  Saturation/1 -> discrete filter/1
  discrete filter/1 -> Sum/2, Sum2/2
  p0/1 -> Sum2/1
  in_1/1 -> Sum/1
  Sum2/1 -> yV/1

== system libc_parts_valves/Ventilsimulation (Zweikanal)/Durchflussfunktion 2-Kanal (sim) ==
  pH : Inport
  p : Inport  Port=2
  pL : Inport  Port=3
  bHbL : Inport  Port=4
  Durchflussfunktion 2 : MATLAB Function  TreatAsAtomicUnit=on
      settings: AttributesFormatString=Wurzelfunktion
  PsiP_bel : Outport
  PsiP_ent : Outport  Port=2
  wires:
  pH/1 -> Durchflussfunktion 2/1(pH)
  pL/1 -> Durchflussfunktion 2/3(pL)
  p/1 -> Durchflussfunktion 2/2(p)
  bHbL/1 -> Durchflussfunktion 2/4(bHbL)
  Durchflussfunktion 2/1(PsiP_bel) -> PsiP_bel/1
  Durchflussfunktion 2/2(PsiP_ent) -> PsiP_ent/1

== matlab function libc_parts_valves/Durchflussfunktion 2-Kanal <alt>/Durchflussfunktion 2 ==
  data: isBel input; pV input; p input; PsiP output; pE input; aVaEcVcE input
function PsiP  = PsiP(isBel, pV, p, pE, aVaEcVcE)
%#codegen
    aV = aVaEcVcE(1);
    aE = aVaEcVcE(2);
    cV = aVaEcVcE(3);
    cE = aVaEcVcE(4);
    
    PsiP_bel = aV*(pV-p)./(cV*pV-p) .* pV;
    PsiP_ent = aE*(p-pE)./(cE*p-pE) .* p;

    PsiP = isBel*PsiP_bel + (1-isBel)*PsiP_ent;
end

== matlab function libc_parts_valves/Durchflussfunktion 2-Kanal/Durchflussfunktion 2 ==
  data: pH input; p input; PsiP_bel output; pL input; aHaLcHcL input; PsiP_ent output
function [PsiP_bel, PsiP_ent] = PsiP(pH, p, pL, aHaLcHcL)
%#codegen
    aH = aHaLcHcL(1);
    aL = aHaLcHcL(2);
    cH = aHaLcHcL(3);
    cL = aHaLcHcL(4);
    
    PsiP_bel = aH*(pH-p)./(cH*pH-p) .* pH;
    PsiP_ent = aL*(p-pL)./(cL*p-pL) .* p;
end

== matlab function libc_parts_valves/Leitwert (erweitert)/InvertInterpolation ==
  data: u_lt input; y_lt input; u input; y output; y_offset input
function y = interpolation(u_lt, y_lt, u, y_offset)
%#codegen

%% Neue Version

y = interp1(u_lt, y_lt, u,'linear','extrap') + y_offset;

%% Alte, PLC-kompatible Version
% ursprünglich für invertierte Interpolation geschrieben, 
% daher müssten y und u vertauscht werden (Berechnung von u(y) statt y(u))

% maxIndex = length(u_lt);
% wert = 0;
% lauf = 0;
% 
% if y <= y_lt(1)
%     % keine Extrapolation
%     wert = u_lt(1);
% elseif y < y_lt(maxIndex)
%     for bpIndex = 1:1:maxIndex
%         if y <= y_lt(bpIndex) && lauf == 0
%             lauf = 1;
%             iRight = bpIndex;
%             iLeft = bpIndex - 1;
%             steig = ((u_lt(iRight) - u_lt(iLeft))/(y_lt(iRight) - y_lt(iLeft)));
%             b = u_lt(iRight) - steig * y_lt(iRight); % lineare Interpolation
%             wert = steig * y + b;
%         end
%     end
% else
%     % keine Extrapolation
%     wert = u_lt(maxIndex);
% end
% u = wert + offset;

== matlab function libc_parts_valves/Leitwert/Invertierung? ==
  data: isinvert input; y input; u input; y_out output; u_out output; sign_out output
function [y_out, u_out, sign_out]  = invert(isinvert, y, u)
%#codegen

if isinvert
    y_out = y;
    u_out = u;
    sign_out = 1;
else
    y_out = u;
    u_out = y;
    sign_out = -1;
end

== matlab function libc_parts_valves/Durchflussfunktion MPYE/limit_pL_14 ==
  data: pHigh input; pSek output; pLow input
function pSek = limp(pHigh, pLow)
    
    %% Weicher Schalter für Druckniveau. 
    % Sekundärdruck wird an Primärdruck angepasst, sodass keine negative
    % Druckdifferenz entstehen kann und somit Psi stets >=1 ist.
    softswitch = tanh(pHigh-pLow)/2+0.5;
    pSek = pLow.*softswitch + (1-softswitch).*pHigh;    

return

== matlab function libc_parts_valves/Durchflussfunktion MPYE/limit_pL_1 ==
  data: pHigh input; pSek output; pLow input
function pSek = limp(pHigh, pLow)
    
    %% Weicher Schalter für Druckniveau. 
    % Sekundärdruck wird an Primärdruck angepasst, sodass keine negative
    % Druckdifferenz entstehen kann und somit Psi stets >=1 ist.
    softswitch = tanh(pHigh-pLow)/2+0.5;
    pSek = pLow.*softswitch + (1-softswitch).*pHigh;    

return

== matlab function libc_parts_valves/Leitwert (erweitert)/Invertierung? ==
  data: u_out output; isinvert input; C input; offset input; u input; y_out output; u_offset output; y_offset output
function [u_out, y_out, u_offset, y_offset]  = invert(isinvert, C, offset, u) 
%#codegen

%% Bemerkungen zur aktuellen Offset-Implementierung
%  positiver u-Offset bedeutet: 
%       bei u=0 wird bereits Belüftet, d.h. Cn(u) ist nach links verschoben
%       Implementierung: Vorwärtsrechnung: kein y-Offset, neg. u-Offset
%                        Invertierung:     neg. y-Offset, kein u-Offset
%       (Alternative):   Vorwärtsrechnung: pos. y-Offset, kein u-Offset
%       |                Invertierung:     kein y-Offset, pos. u-Offset
%       (bei u=0 wird bereits Belüftet, d.h. Cn(u) ist nach oben verschoben
%
%  alternative Interpretation (hier nicht verwendet):
%       man muss einen positiven Offset verwenden,
%       um bei u=0 nicht mehr zu Belüften.
%
% ! PLC Code (deaktiviert): Offset negativ (anderes) definiert

%% Funktion

if ~isinvert
    % Vorwärtsberechnung. 
    % Eingänge werden nicht vertauscht, da später Interpolation y_out=lt(u_out)
    % Cn = Cn(u + offset);
    y_out = C;
    u_out = u;
    %y_offset = 0;
    %u_offset = -offset;
    y_offset = -offset;
    u_offset = 0;
else
    % Modellinvertierung. 
    % Eingänge werden vertauscht, da später Interpolation y_out=lt(u_out)
    % u = u(Cinv) + offset;
    y_out = u;
    u_out = C;
    %y_offset = -offset;
    %u_offset = 0;
    y_offset = 0;
    u_offset = -offset;
end

% nächster Block: y_out = interp1(lty, ltu, u_out + u_offset) + y_offset

== matlab function libc_parts_valves/Leitwert (erweitert)/Lookuptabelle initialisieren/Initialize LookupTable ==
  data: Cn14_safe output; Cn45_safe output; shapewarning output; Cn14 output; Cn45 output; pfcf input; pm1 input; pm2 input; pxue input; prund input; pleck input; u output; pdelle input; pxue2 input; pabsk input; pshape input
function [Cn14_safe, Cn45_safe, shapewarning, Cn14, Cn45, u] = int_abs(pfcf, pm1, pm2, pxue, prund ,pleck, pdelle, pxue2, pabsk, pshape)
%#codegen

%% Ordinate: Variable Schrittweite
% gleiche Parameter für negativen Zweig
mxue = pxue;

% Datenpunkte: n = 2*n_grob + n_fein
%n_grob = 25;n_fein = 50;
n_grob = 10;n_fein = 30;
%n_grob = 10;n_fein = 10;
u=[linspace(-1,-mxue*1.2,n_grob),linspace(-mxue*1.18,pxue*1.18,n_fein),linspace(pxue*1.2,1,n_grob)];

%% Ordinate: Alte, feste Schrittweite
%u=[(-1:0.1:-0.2),(-0.18:0.02:0.18),(0.2:0.1:1.0)];


%% Abszisse: Neue, schnelle Version

% gleiche Parameter für negativen Zweig
mfcf = pfcf;
mm1  = pm1;
mm2  = pm2;
mxue = pxue;
mrund = prund;
mleck = pleck;

% auch für neue Parameter
mdelle = pdelle;
mxue2 = pxue2;
mabsk = pabsk;
mshape = pshape;

% Grundversion
pC_ges = ((pm2-pm1)*pxue-pm2-pleck)^(-3) + pfcf^(-3);
mC_ges = ((mm2-mm1)*mxue-mm2-mleck)^(-3) + mfcf^(-3);
refit_c_14 = ((pm1*  u  + (pm2-pm1)*prund*(tanh(( u-pxue)/prund-1)+1)+pleck) .* ((-pleck/pm1<= u)& ( u<pxue+prund)) + (abs((pm2*  u  + (pm1-pm2)*pxue+pleck).^(-3) + pC_ges )).^(-1/3) .* ( u>=pxue+prund));
refit_c_45 = ((mm1*(-u) + (mm2-mm1)*mrund*(tanh((-u-mxue)/mrund-1)+1)+mleck) .* ( -mleck/mm1<=-u).*(-u<mxue+mrund)  + (abs((mm2*(-u) + (mm1-mm2)*mxue+mleck).^(-3) + mC_ges )).^(-1/3) .* (-u>=mxue+mrund));

% Erweiterung: neuer shapefix (deaktiviert bei ungünstigen Parametern)
shapewarning = 0;
if (pdelle == 0) || (pabsk == 0) || (pdelle <= pxue) || (pxue2 <= pdelle) 
    shapefix_14 = u*0;
else
    shapefix_14   = pabsk*((0.5*cos(( u-pdelle)./((pdelle-pxue)*( u<=pdelle) + (pxue2-pdelle)*( u>pdelle))*pi)+0.5).*(1-pshape) + pshape.*(0.5*cos((( u-pdelle)./((pdelle-pxue)*( u<=pdelle) + (pxue2-pdelle)*( u>pdelle))).^3*pi)+0.5)).*(( u>=pxue)&( u<pxue2));
    cleardiffdata = max(diff(shapefix_14),-diff(refit_c_14));
    if sum(abs(diff(shapefix_14)-cleardiffdata)) > 0
        shapefix_14   = cumsum([0 cleardiffdata].*u);
        shapewarning = 1;
    end
end
if (mdelle == 0) || (mabsk == 0) || (mdelle <= mxue) || (mxue2 <= mdelle) 
    shapefix_45 = u*0;
else
    shapefix_45   = mabsk*((0.5*cos((-u-mdelle)./((mdelle-mxue)*(-u<=mdelle) + (mxue2-mdelle)*(-u>mdelle))*pi)+0.5).*(1-mshape) + mshape.*(0.5*cos(((-u-mdelle)./((mdelle-mxue)*(-u<=mdelle) + (mxue2-mdelle)*(-u>mdelle))).^3*pi)+0.5)).*((-u>=mxue)&(-u<mxue2));
    cleardiffdata = max(diff(fliplr(shapefix_45)),-diff(fliplr(refit_c_45)));
    if sum(abs(diff(fliplr(shapefix_45))-cleardiffdata)) > 0
        shapefix_45   = fliplr(cumsum([0 cleardiffdata].*u));
        shapewarning = 1;
    end
end


Cn14 = refit_c_14 + shapefix_14;
Cn45 = refit_c_45 - shapefix_45;
Cn14_safe = refit_c_14;
Cn45_safe = refit_c_45;

%% Abszisse: Alte, kompatible Version (PLC)
% ohne Leckstrom/Leckage
% ohne Erweiterung

% C_ges_hm3= ((pm2-pm1)*pxue-pm2)^(-3) + pfcf^(-3);
% 
% C = u;
% for lauf = 1:length(u)
%    if abs(u(lauf)) >= (pxue+prund)
%        C(lauf) = ((pm2*abs(u(lauf)) + (pm1-pm2)*pxue)^(-3) + C_ges_hm3 )^(-1/3);
%    else
%        C(lauf) = (pm1*abs(u(lauf)) + (pm2-pm1)*prund*(1-2/(exp(((abs(u(lauf))-pxue)/prund-1))+1)+1));
%    end
% end
% 
% % alte, falsche Funktion
% C =(C).*abs(u+1e-9)./(u+1e-9)/pfcf;
% % alte, korrigierte Funktion
% C =(C).*abs(u+1e-9)./(u+1e-9);

end

== matlab function libc_parts_valves/Durchflussfunktion 2-Kanal (sim)/Durchflussfunktion 2 ==
  data: pH input; p input; PsiP_bel output; pL input; bHbL input; PsiP_ent output
function [PsiP_bel, PsiP_ent] = PsiP(pH, p, pL, bHbL)
%#codegen    

    b_bel = bHbL(1);
    b_ent = bHbL(2);
    
    PsiP_bel = sqrt(1-((max(min(1,p./pH),b_bel)-b_ent)/(1-b_bel)).^2) .* pH;
    PsiP_ent = sqrt(1-((max(min(1,pL./p),b_ent)-b_ent)/(1-b_ent)).^2) .* p;
end

== matlab function libc_parts_valves/Leitwert Knickfunktion ==
  data: u input; C output; knick_u input; knick_C input
function C = knick(u, knick_u, knick_C) 
% für Rückwärtstransformation einfach 
%   * u und C vertauschen (I<-->O)
%   * knick_u und knick_C vertauschen
%#codegen


m1 = knick_C./knick_u;
m2 = (1-knick_C)./(1-knick_u);
o2 = knick_C - (1-knick_C)./(1-knick_u).*knick_u;

C = (m1.*u).*(knick_u>=u) + (m2.*u+o2).*(knick_u<u);

== matlab function libc_parts_valves/Durchflussfunktion 1-Kanal/Durchflussfunktion 1 ==
  data: pPrim input; pSek input; a input; c input; PsiP output
function PsiP = PsiP(pPrim, pSek, a, c)

    % Durchflussfunktion mit Primärdruck
    PsiP = a*(pPrim - pSek)./(c*pPrim - pSek) .* pPrim;   

return

== matlab function libc_parts_valves/Massenstrom/Massenstrom ==
  data: parrho input; parC input; parb input; pBefore input; mBdot output; pAfter input
function mBdot = mB(parrho, parC, parb, pBefore, pAfter)


    %% Parameter (ext)

    %c0 = 1.07+(0.6-parb)*0.2;  % Faustformel für c-Wert der gebrochen-rationalen Funktion, für b e (0.2,0.55)
    %a1 = (c0 - parb/2)./(1 - parb/2);   % Faktor 1/2 ist Fummelfaktor, um den Sqrt-b-Wert sinnvoll zu verwenden (Skalierung von "normalem" b-Wert (sqrt) zu angepasstem b-Wert (gebrochen-rationale Fkt))
    %a2 = a1;
    
    % Approximierte Durchflussfunktion bei kritischem Druckverhältnis,
    % Näherungsformel aus D:\Dokumente\Tools\Matlab_FestoLib\psi_param.m
    [a1, a2, c0] = psi_param(parb);

    %% Weicher Schalter für Druckniveau. 
    % Sekundärdruck wird an Primärdruck angepasst, sodass keine negative
    % Druckdifferenz entstehen kann und somit Psi stets >=1 ist.
    softswitch = tanh(pBefore-pAfter)/2+0.5;
    pMin = pAfter.*softswitch + (1-softswitch).*pBefore; % ~ min(pAfter,pBefore)
    
    %% Gebrochenrationale Psi-Funktion
    % Diese Durchflussfunktion hat keine unendliche Steigung im
    % Gleichgewichtspunkt. 
    % In dieser speziellen Form wird nicht Psi sondern Psi*pprim berechnet
    PsiPP = a1.*(pBefore-pMin)./(c0 - pMin./pBefore);
    PsiPN = a2.*(pAfter -pMin)./(c0 - pMin./pAfter );
    
    %% Wurzelfunktion für Psi (steilerer Nulldurchgang bei Massenfluss)
    %PsiPP = pBefore.*sqrt((1-(tanh((pMin./pBefore-parb-0.001)*1000)/2+0.5).*((pMin./pBefore-parb)./(1-parb)).^2));
    %PsiPN = pAfter.* sqrt((1-(tanh((pMin./pAfter -parb-0.001)*1000)/2+0.5).*((pMin./pAfter -parb)./(1-parb)).^2));
    
    %% Gesamter Massenstrom als Differenz
    mBdot = parrho*parC.*(PsiPP - PsiPN);
    
    %% Debug

    % M = [mBdotIn; mBdotOut];
    % P = [PsiIn; PsiOut];
    % Q = [qIn; qOut];
    
end

== matlab function libc_parts_valves/Leitwert/InvertInterpolation ==
  data: y_lt input; u_lt input; offset input; Cn input; u output
function u = interpolation(y_lt, u_lt, offset, Cn)
%#codegen

%% Neue Version

u = interp1(y_lt, u_lt, Cn,'linear','extrap') + offset;

%% Alte, PLC-kompatible Version

% maxIndex = length(u_lt);
% wert = 0;
% lauf = 0;
% 
% if Cn <= y_lt(1)
%     % keine Extrapolation
%     wert = u_lt(1);
% elseif Cn < y_lt(maxIndex)
%     for bpIndex = 1:1:maxIndex
%         if Cn <= y_lt(bpIndex) && lauf == 0
%             lauf = 1;
%             iRight = bpIndex;
%             iLeft = bpIndex - 1;
%             steig = ((u_lt(iRight) - u_lt(iLeft))/(y_lt(iRight) - y_lt(iLeft)));
%             b = u_lt(iRight) - steig * y_lt(iRight); % lineare Interpolation
%             wert = steig * Cn + b;
%         end
%     end
% else
%     % keine Extrapolation
%     wert = u_lt(maxIndex);
% end
% u = wert + offset;

== matlab function libc_parts_valves/Leitwert/Lookuptabelle initialisieren/Initialize LookupTable ==
  data: pfcf input; pm1 input; pm2 input; pxue input; prund input; pleck input; y output; u output
function [y, u] = int_abs(pfcf,pm1,pm2,pxue,prund,pleck)
%#codegen

%% Ordinate: Variable Schrittweite
mxue = pxue;

% Datenpunkte: n = 2*n_grob + n_fein
n_grob = 10;
n_fein = 20;

u=[linspace(-1,-mxue*1.2,n_grob),linspace(-mxue*1.1,pxue*1.1,n_fein),linspace(pxue*1.2,1,n_grob)];

%% Ordinate: Alte, feste Schrittweite
%u=[(-1:0.1:-0.2),(-0.18:0.02:0.18),(0.2:0.1:1.0)];



%% Abszisse: Neue, schnelle Version

mfcf = pfcf;
mm1  = pm1;
mm2  = pm2;
mxue = pxue;
mrund = prund;
mleck = pleck;

pC_ges = ((pm2-pm1)*pxue-pm2-pleck)^(-3) + pfcf^(-3);
mC_ges = ((mm2-mm1)*mxue-mm2-mleck)^(-3) + mfcf^(-3);

refit_c_14 = ((pm1*  u  + (pm2-pm1)*prund*(tanh(( u-pxue)/prund-1)+1)+pleck) .* ((-pleck/pm1<=u )& ( u<pxue+prund)) + (abs((pm2*  u  + (pm1-pm2)*pxue+pleck).^(-3) + pC_ges )).^(-1/3) .* ( u>=pxue+prund));
refit_c_45 = ((mm1*(-u) + (mm2-mm1)*mrund*(tanh((-u-mxue)/mrund-1)+1)+mleck) .* ( -mleck/mm1<=-u).*(-u<mxue+mrund)  + (abs((mm2*(-u) + (mm1-mm2)*mxue+mleck).^(-3) + mC_ges )).^(-1/3) .* (-u>=mxue+mrund));

y = refit_c_14 - refit_c_45;

%% Abszisse: Alte, kompatible Version (PLC)
% ohne Leckstrom/Leckage

% C_ges_hm3= ((pm2-pm1)*pxue-pm2)^(-3) + pfcf^(-3);
% 
% y = u;
% for lauf = 1:length(u)
%    if abs(u(lauf)) >= (pxue+prund)
%        y(lauf) = ((pm2*abs(u(lauf)) + (pm1-pm2)*pxue)^(-3) + C_ges_hm3 )^(-1/3);
%    else
%        y(lauf) = (pm1*abs(u(lauf)) + (pm2-pm1)*prund*(1-2/(exp(((abs(u(lauf))-pxue)/prund-1))+1)+1));
%    end
% end
% 
% % alte, falsche Funktion
% y =(y).*abs(u+1e-9)./(u+1e-9)/pfcf;
% % alte, korrigierte Funktion
% y =(y).*abs(u+1e-9)./(u+1e-9);

end

== matlab function libc_parts_valves/Reine Durchflussfunktion 2-Kanal (sim)/Durchflussfunktion 2 ==
  data: pH input; p input; Psi_bel output; pL input; bHbL input; Psi_ent output
function [Psi_bel, Psi_ent] = PsiP(pH, p, pL, bHbL)
%#codegen    

    b_bel = bHbL(1);
    b_ent = bHbL(2);
    
    Psi_bel = sqrt(1-((max(min(1,p./pH),b_bel)-b_ent)/(1-b_bel)).^2);
    Psi_ent = sqrt(1-((max(min(1,pL./p),b_ent)-b_ent)/(1-b_ent)).^2);
end

== matlab function libc_parts_valves/Ventilsimulation (Zweikanal)/Durchflussfunktion 2-Kanal (sim)/Durchflussfunktion 2 ==
  data: pH input; p input; PsiP_bel output; pL input; bHbL input; PsiP_ent output
function [PsiP_bel, PsiP_ent] = PsiP(pH, p, pL, bHbL)
%#codegen    

    b_bel = bHbL(1);
    b_ent = bHbL(2);
    
    PsiP_bel = sqrt(1-((max(min(1,p./pH),b_bel)-b_ent)/(1-b_bel)).^2) .* pH;
    PsiP_ent = sqrt(1-((max(min(1,pL./p),b_ent)-b_ent)/(1-b_ent)).^2) .* p;
end

== matlab function libc_parts_valves/Psi Param/b-auto ==
  data: b input; a1 output; a2 output; c0 output
function [a1,a2,c0]  = sqrt2gebrat(b)
%#codegen

    [a1,a2,c0] = psi_param(b);

end

== matlab function libc_parts_valves/Ventilsimulation (Einkanal)/soft-switch-enabled ==
  data: Cbel input; C output; alpha input; Cent input
function C = s(Cbel, alpha, Cent)
%#codegen

C = Cbel.*alpha + (1-alpha).*Cent;
